simulink model "orden1_sim"  (R2025a)
settings: Solver=FixedStepAuto  StartTime=0.0  StopTime=30.0  FixedStep=0.01  RelTol=1e-3
values from neighbouring files (symbols this model uses):
  Kp = (2*xi_m*Tm1)/(K*L) * (1 - 1/Ms)    [diseno_controladores.m]    (also in orden1_controladores.m = (T + 0.5*L) / (K * (lambda + L)))
  L = 0.089649500000000    (= 0.0896495)    [diseno_controladores.m]    (also in orden1_controladores.m = 0.1371)
  P_nodelay = K/(T*s+1)    [orden1_controladores.m]
  Td = Tm1/(2*xi_m)    [diseno_controladores.m]    (also in orden1_controladores.m = 0.0643515613134)
  Ti = 2*xi_m*Tm1    [diseno_controladores.m]    (also in orden1_controladores.m = 1.11925)
  Ts = 0.0265    [orden1_controladores.m]
undefined symbols (not defined in the file or in its folder): D, uDelay, xinit, yDelay
libraries: cstblocks x2
settings Model: Creator=danielsaenzobando  LastModifiedBy=danielsaenzobando

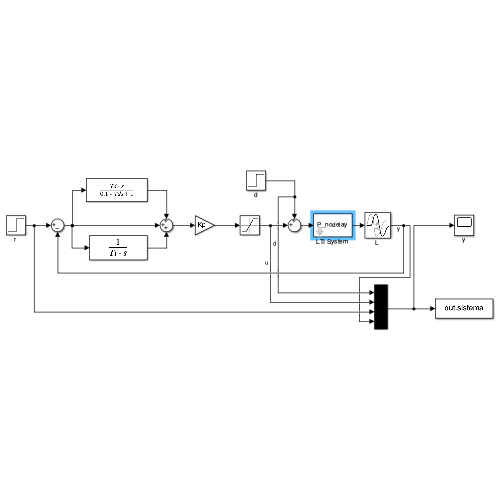
[thumbnail: Simulink's stored preview of the top-level diagram]
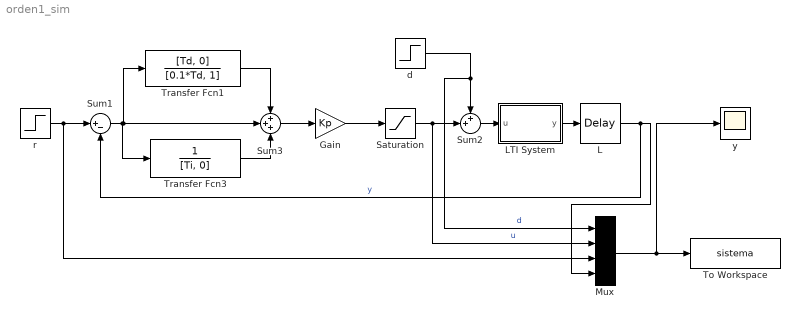
== system orden1_sim ==
  Gain : Gain  Gain=Kp
  L : TransportDelay  DelayTime=L  BufferSize=2048  FixedBuffer=on
  LTI System : Subsystem  BlockChoice=CSS  mask(LTI Block){sys=P_nodelay, IC=[], PadeOrder=0}
      mask prompts: sys "Control:simulink:LTIMaskLabel1"; IC "Control:simulink:LTIMaskLabel2"; PadeOrder "Pade Order (for linearization)"
      mask help: Control:simulink:LTIMaskDescription
      mask init:
      | model = bdroot;
      | df = get_param(model,'dirty');
      | try
      |     [D,uDelay,yDelay,xinit,Ts,sysname] = controllib.internal.blocks.lti.ltimaskData(gcb,sys,IC);
      | catch ME
      |     sysname = '???';
      |     throwAsCaller(MSLException(get_param(gcb,'handle'),ME.identifier,ME.message))
      | end
      | controllib.internal.blocks.lti.ltimaskUpdate(gcb,D,xinit,Ts,PadeOrder)
      | try
      |     % Attempt to modify locked library -> error
      |     set_param(model,'dirty',df)
      | end
      mask Help: eval('helpview(''control'',''ltisystemblock'');')
      mask Callback sys: controllib.internal.blocks.lti.ltimaskCallback(gcb,'System')
      mask DialogControl sys Prompt: LTI system variable
      mask DialogControl IC Prompt: Initial states (state-space only)
      mask Display: disp(sysname)
  Mux : Mux
  Saturation : Saturate  UpperLimit=100  LowerLimit=0
  Sum1 : Sum  Inputs=|+-
  Sum2 : Sum  Inputs=++|
  Sum3 : Sum  Inputs=+++
  To Workspace : ToWorkspace  VariableName=sistema  SaveFormat=Timeseries  SampleTime=-1
  Transfer Fcn1 : TransferFcn  Numerator=[Td, 0]  Denominator=[0.1*Td, 1]
  Transfer Fcn3 : TransferFcn  Denominator=[Ti, 0]
  d : Step  Time=20  After=10  SampleTime=0
  "r " : Step  Time=5  After=20  SampleTime=0
  y : Scope
      settings: ActiveDisplayYMinimum=-39.063047037354828  ActiveDisplayYMaximum=135.53887336337169
  wires:
  Sum2/1 -> LTI System/1(u)
  Mux/1 -> y/1, To Workspace/1
  L/1 -> Mux/4, Sum1/2  "y"
  "r "/1 -> Mux/3, Sum1/1
  Sum1/1 -> Sum3/2, Transfer Fcn1/1, Transfer Fcn3/1
  LTI System/1(y) -> L/1
  Gain/1 -> Saturation/1
  Sum3/1 -> Gain/1
  Transfer Fcn1/1 -> Sum3/1
  Transfer Fcn3/1 -> Sum3/3
  Saturation/1 -> Sum2/2, Mux/2  "u"
  d/1 -> Sum2/1, Mux/1  "d"

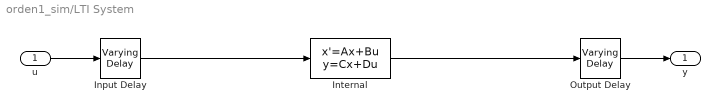
== system orden1_sim/LTI System ==
  u : Inport  PortDimensions=1  SampleTime=Ts
  Input Delay : cstblocks/Linear Parameter Varying/Varying Delay  Td=uDelay  TdMax=max(uDelay)  TdMin=0  TdFixed=1  u0=0  bufsize=1024  FixedBuffer=off  PadeOrder=0
  Internal : StateSpace  A=D.a  B=D.b  C=D.c  D=D.d  InitialCondition=xinit
  Output Delay : cstblocks/Linear Parameter Varying/Varying Delay  Td=yDelay  TdMax=max(yDelay)  TdMin=0  TdFixed=1  u0=0  bufsize=1024  FixedBuffer=off  PadeOrder=0
  y : Outport  InitialOutput=0  VectorParamsAs1DForOutWhenUnconnected=off
  wires:
  u/1 -> Input Delay/1
  Output Delay/1 -> y/1
  Input Delay/1 -> Internal/1
  Internal/1 -> Output Delay/1
